simulink model "EMC_no_hand"  (R2015a)
settings: Solver=ode4  SolverMode=MultiTasking  StartTime=0.0  StopTime=inf  FixedStep=BKIN_STEP_TIME  RelTol=1e-3
StartFcn:
  |  warndlg('Dexterit-E models cannot run under simulation. Please compile your model and run it from within Dexterit-E.');set_param(bdroot,'SimulationCommand','stop')
model workspace (MAT data in the model file):
  BKIN_KINEMATIC_FRAME_SIZE = 400
  BKIN_STEP_TIME = 0.00025
  COLOR = 4
  COL_X = 1
  COL_Y = 2
  E_NO_EVENT = 0
  LOAD_X = 1
  LOAD_Y = 2
  MOVEMENT_DELAY = 3
  PATH_LENGTH = 1
  PATH_PERIOD = 2
  POST_TRIAL_DELAY = 4
  RADIUS = 3
  TRAJECTORY = 1
  TRAJECTORY_TYPE = 2
  TRIAL_END = 3
  TRIAL_MOVEMENT = 2
  TRIAL_RESET = 4
  TRIAL_START = 1
  X_POSITION = 1
  Y_POSITION = 2
  col_x = 1
  col_y = 2
  ANGULAR_THRESHOLD = 5
  GAZE_EXIT = 6
  START_REACHED = 7
  FIXATION_DURATION = 6
  TRACKING_TARGET_ROW = 7
  FEEDBACK_COLOR = 5
  CROSS_LOGICAL_RADIUS = 8
  DETECT_FIXATION = 8
  GAZE_IN_TARGET = 5
  START_STABILIZATION = 9
  HAND_IN_TARGET = 9
  BACKGROUND_LOAD = 10
  DIST_BETWEEN_TRAJ = 11
  STRAIGHT_PAUSE_TIME = 12
libraries: simulink x14, xpcrtudplib x12, xpcutilitieslib x10, xpcobsoletelib x8, slrtlib x2, ethercat x2, General x2, Video x2
(part 3 of 6)

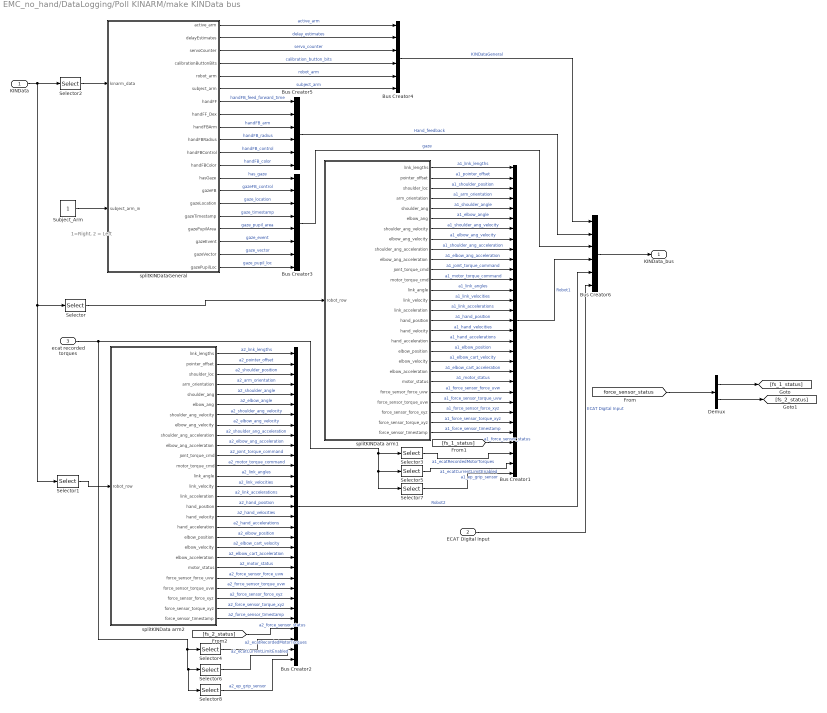
== system EMC_no_hand/DataLogging/Poll KINARM/make KINData bus ==
  note: 1=Right, 2 = Left
  KINData : Inport
  ECAT Digital Input : Inport  Port=2
  ecat recorded torques : Inport  Port=3
  Bus Creator1 : BusCreator  Inputs=31
  Bus Creator2 : BusCreator  Inputs=31
  Bus Creator3 : BusCreator  Inputs=8
  Bus Creator4 : BusCreator  Inputs=6
  Bus Creator5 : BusCreator  Inputs=6
  Bus Creator6 : BusCreator  Inputs=6
  Demux : Demux  Outputs=2
  Selector : Selector  NumberOfDimensions=2  InputPortWidth=3  IndexOptions=Index vector (dialog),Select all  Indices=[1],1  OutputSizes=1,1
  Selector1 : Selector  NumberOfDimensions=2  InputPortWidth=3  IndexOptions=Index vector (dialog),Select all  Indices=[2],1  OutputSizes=1,1
  Selector2 : Selector  NumberOfDimensions=2  InputPortWidth=3  IndexOptions=Index vector (dialog),Select all  Indices=[3],1  OutputSizes=1,1
  Selector3 : Selector  Indices=[1 2]
  Selector4 : Selector  Indices=[3, 4]
  Selector5 : Selector  Indices=[5 6]
  Selector6 : Selector  Indices=[7, 8]
  Selector7 : Selector  Indices=[9]
  Selector8 : Selector  Indices=[10]
  Subject_Arm : Constant
  splitKINData arm1 : MATLAB Function  TreatAsAtomicUnit=on
  splitKINData arm2 : MATLAB Function  TreatAsAtomicUnit=on
  splitKINDataGeneral : MATLAB Function  TreatAsAtomicUnit=on
  KINData_bus : Outport
  wires:
  splitKINDataGeneral/20(gazePupilLoc) -> Bus Creator3/8  "gaze_pupil_loc"
  splitKINDataGeneral/13(hasGaze) -> Bus Creator3/1  "has_gaze"
  splitKINDataGeneral/14(gazeFB) -> Bus Creator3/2  "gazeFB_control"
  splitKINDataGeneral/15(gazeLocation) -> Bus Creator3/3  "gaze_location"
  splitKINDataGeneral/16(gazeTimestamp) -> Bus Creator3/4  "gaze_timestamp"
  splitKINDataGeneral/17(gazePupilArea) -> Bus Creator3/5  "gaze_pupil_area"
  splitKINDataGeneral/18(gazeEvent) -> Bus Creator3/6  "gaze_event"
  splitKINData arm1/1(link_lengths) -> Bus Creator1/1  "a1_link_lengths"
  splitKINData arm1/2(pointer_offset) -> Bus Creator1/2  "a1_pointer_offset"
  splitKINData arm1/3(shoulder_loc) -> Bus Creator1/3  "a1_shoulder_position"
  splitKINData arm1/4(arm_orientation) -> Bus Creator1/4  "a1_arm_orientation"
  splitKINData arm1/5(shoulder_ang) -> Bus Creator1/5  "a1_shoulder_angle"
  splitKINData arm1/6(elbow_ang) -> Bus Creator1/6  "a1_elbow_angle"
  splitKINData arm1/7(shoulder_ang_velocity) -> Bus Creator1/7  "a1_shoulder_ang_velocity"
  splitKINData arm1/8(elbow_ang_velocity) -> Bus Creator1/8  "a1_elbow_ang_velocity"
  splitKINData arm1/11(joint_torque_cmd) -> Bus Creator1/11  "a1_joint_torque_command"
  splitKINData arm1/12(motor_torque_cmd) -> Bus Creator1/12  "a1_motor_torque_command"
  splitKINData arm1/13(link_angle) -> Bus Creator1/13  "a1_link_angles"
  splitKINData arm1/14(link_velocity) -> Bus Creator1/14  "a1_link_velocities"
  splitKINData arm1/15(link_acceleration) -> Bus Creator1/15  "a1_link_accelerations"
  splitKINData arm1/16(hand_position) -> Bus Creator1/16  "a1_hand_position"
  splitKINData arm1/17(hand_velocity) -> Bus Creator1/17  "a1_hand_velocities"
  splitKINData arm1/18(hand_acceleration) -> Bus Creator1/18  "a1_hand_accelerations"
  splitKINData arm1/22(motor_status) -> Bus Creator1/22  "a1_motor_status"
  splitKINData arm1/23(force_sensor_force_uvw) -> Bus Creator1/23  "a1_force_sensor_force_uvw"
  splitKINData arm1/24(force_sensor_torque_uvw) -> Bus Creator1/24  "a1_force_sensor_torque_uvw"
  splitKINData arm1/25(force_sensor_force_xyz) -> Bus Creator1/25  "a1_force_sensor_force_xyz"
  splitKINData arm1/26(force_sensor_torque_xyz) -> Bus Creator1/26  "a1_force_sensor_torque_xyz"
  splitKINData arm1/27(force_sensor_timestamp) -> Bus Creator1/27  "a1_force_sensor_timestamp"
  splitKINData arm2/1(link_lengths) -> Bus Creator2/1  "a2_link_lengths"
  splitKINData arm2/2(pointer_offset) -> Bus Creator2/2  "a2_pointer_offset"
  splitKINData arm2/3(shoulder_loc) -> Bus Creator2/3  "a2_shoulder_position"
  splitKINData arm2/4(arm_orientation) -> Bus Creator2/4  "a2_arm_orientation"
  splitKINData arm2/5(shoulder_ang) -> Bus Creator2/5  "a2_shoulder_angle"
  splitKINData arm2/6(elbow_ang) -> Bus Creator2/6  "a2_elbow_angle"
  splitKINData arm2/7(shoulder_ang_velocity) -> Bus Creator2/7  "a2_shoulder_ang_velocity"
  splitKINData arm2/11(joint_torque_cmd) -> Bus Creator2/11  "a2_joint_torque_command"
  splitKINData arm2/12(motor_torque_cmd) -> Bus Creator2/12  "a2_motor_torque_command"
  splitKINData arm2/13(link_angle) -> Bus Creator2/13  "a2_link_angles"
  splitKINData arm2/14(link_velocity) -> Bus Creator2/14  "a2_link_velocities"
  splitKINData arm2/15(link_acceleration) -> Bus Creator2/15  "a2_link_accelerations"
  splitKINData arm2/16(hand_position) -> Bus Creator2/16  "a2_hand_position"
  splitKINData arm2/17(hand_velocity) -> Bus Creator2/17  "a2_hand_velocities"
  splitKINData arm2/18(hand_acceleration) -> Bus Creator2/18  "a2_hand_accelerations"
  splitKINData arm2/22(motor_status) -> Bus Creator2/22  "a2_motor_status"
  splitKINData arm2/23(force_sensor_force_uvw) -> Bus Creator2/23  "a2_force_sensor_force_uvw"
  splitKINData arm2/24(force_sensor_torque_uvw) -> Bus Creator2/24  "a2_force_sensor_torque_uvw"
  splitKINData arm2/25(force_sensor_force_xyz) -> Bus Creator2/25  "a2_force_sensor_force_xyz"
  splitKINData arm2/26(force_sensor_torque_xyz) -> Bus Creator2/26  "a2_force_sensor_torque_xyz"
  splitKINData arm2/27(force_sensor_timestamp) -> Bus Creator2/27  "a2_force_sensor_timestamp"
  Selector/1 -> splitKINData arm1/1(robot_row)
  Selector1/1 -> splitKINData arm2/1(robot_row)
  splitKINDataGeneral/1(active_arm) -> Bus Creator4/1  "active_arm"
  splitKINDataGeneral/2(delayEstimates) -> Bus Creator4/2  "delay_estimates"
  splitKINDataGeneral/3(servoCounter) -> Bus Creator4/3  "servo_counter"
  splitKINDataGeneral/4(calibrationButtonBits) -> Bus Creator4/4  "calibration_button_bits"
  splitKINDataGeneral/7(handFF) -> Bus Creator5/1  "handFB_feed_forward_time"
  splitKINDataGeneral/9(handFBArm) -> Bus Creator5/3  "handFB_arm"
  splitKINDataGeneral/10(handFBRadius) -> Bus Creator5/4  "handFB_radius"
  splitKINDataGeneral/11(handFBControl) -> Bus Creator5/5  "handFB_control"
  splitKINDataGeneral/12(handFBColor) -> Bus Creator5/6  "handFB_color"
  Bus Creator4/1 -> Bus Creator6/1  "KINDataGeneral"
  Bus Creator5/1 -> Bus Creator6/2  "Hand_feedback"
  Bus Creator3/1 -> Bus Creator6/3  "gaze"
  Bus Creator1/1 -> Bus Creator6/4  "Robot1"
  Bus Creator2/1 -> Bus Creator6/5  "Robot2"
  KINData/1 -> Selector1/1, Selector/1, Selector2/1
  Bus Creator6/1 -> KINData_bus/1
  Selector2/1 -> splitKINDataGeneral/1(kinarm_data)
  ECAT Digital Input/1 -> Bus Creator6/6  "ECAT Digital Input"
  ecat recorded torques/1 -> Selector7/1, Selector5/1, Selector3/1, Selector4/1, Selector8/1, Selector6/1
  Selector3/1 -> Bus Creator1/29  "a1_ecatRecordedMotorTorques"
  Selector4/1 -> Bus Creator2/29  "a2_ecatRecordedMotorTorques"
  Selector5/1 -> Bus Creator1/30  "a1_ecatCurrentLimitEnabled"
  Selector6/1 -> Bus Creator2/30  "a2_ecatCurrentLimitEnabled"
  splitKINDataGeneral/8(handFF_Dex) -> Bus Creator5/2
  splitKINDataGeneral/19(gazeVector) -> Bus Creator3/7  "gaze_vector"
  [force_sensor_status] -> Demux/1
  Demux/1 -> [fs_1_status]
  Demux/2 -> [fs_2_status]
  [fs_1_status] -> Bus Creator1/28  "a1_force_sensor_status"
  [fs_2_status] -> Bus Creator2/28  "a2_force_sensor_status"
  splitKINData arm1/9(shoulder_ang_acceleration) -> Bus Creator1/9  "a1_shoulder_ang_acceleration"
  splitKINData arm1/10(elbow_ang_acceleration) -> Bus Creator1/10  "a1_elbow_ang_acceleration"
  splitKINData arm1/19(elbow_position) -> Bus Creator1/19  "a1_elbow_position"
  splitKINData arm1/20(elbow_velocity) -> Bus Creator1/20  "a1_elbow_cart_velocity"
  splitKINData arm1/21(elbow_acceleration) -> Bus Creator1/21  "a1_elbow_cart_acceleration"
  splitKINData arm2/10(elbow_ang_acceleration) -> Bus Creator2/10  "a2_elbow_ang_acceleration"
  splitKINData arm2/21(elbow_acceleration) -> Bus Creator2/21  "a2_elbow_cart_acceleration"
  splitKINData arm2/20(elbow_velocity) -> Bus Creator2/20  "a2_elbow_cart_velocity"
  splitKINData arm2/19(elbow_position) -> Bus Creator2/19  "a2_elbow_position"
  splitKINData arm2/8(elbow_ang_velocity) -> Bus Creator2/8  "a2_elbow_ang_velocity"
  splitKINData arm2/9(shoulder_ang_acceleration) -> Bus Creator2/9  "a2_shoulder_ang_acceleration"
  Selector7/1 -> Bus Creator1/31  "a1_ep_grip_sensor"
  Selector8/1 -> Bus Creator2/31  "a2_ep_grip_sensor"
  splitKINDataGeneral/6(subject_arm) -> Bus Creator4/6  "subject_arm"
  splitKINDataGeneral/5(robot_arm) -> Bus Creator4/5  "robot_arm"
  Subject_Arm/1 -> splitKINDataGeneral/2(subject_arm_in)

== system EMC_no_hand/DataLogging/Poll KINARM/split_primary ==
  primary data : Inport
  Bus Creator1 : BusCreator  Inputs=3
  Bus Creator2 : BusCreator  Inputs=2
  Bus Creator4 : BusCreator  Inputs=3
  Selector1 : Selector  NumberOfDimensions=2  InputPortWidth=3  IndexOptions=Index vector (dialog),Select all  Indices=[2],1  OutputSizes=1,1
  Selector2 : Selector  NumberOfDimensions=2  InputPortWidth=3  IndexOptions=Index vector (dialog),Select all  Indices=[1],1  OutputSizes=1,1
  split_primary : MATLAB Function  TreatAsAtomicUnit=on
  split_primary1 : MATLAB Function  TreatAsAtomicUnit=on
  primary_data_bus : Outport
  wires:
  split_primary/1(link_angles) -> Bus Creator4/1  "a1_link_angles"
  split_primary/2(link_velocities) -> Bus Creator4/2  "a1_link_velocities"
  split_primary/3(link_acceleration) -> Bus Creator4/3  "a1_link_accelerations"
  primary data/1 -> Selector2/1, Selector1/1
  Selector2/1 -> split_primary/1(primary_data)
  split_primary1/1(link_angles) -> Bus Creator1/1  "a2_link_angles"
  split_primary1/2(link_velocities) -> Bus Creator1/2  "a2_link_velocities"
  split_primary1/3(link_acceleration) -> Bus Creator1/3  "a2_link_accelerations"
  Selector1/1 -> split_primary1/1(primary_data)
  Bus Creator4/1 -> Bus Creator2/1  "robot1"
  Bus Creator1/1 -> Bus Creator2/2  "robot2"
  Bus Creator2/1 -> primary_data_bus/1

== system EMC_no_hand/DataLogging/apply loads/apply pmac loads ==
  Force scale : Inport
  Torques : Inport  Port=2
  Robot 1 motor parms : Inport  Port=3
  Robot 2 motor parms : Inport  Port=4
  Enable : EnablePort
  Bus Selector : BusSelector  OutputSignals=R1.Arm Orientation,R1.M1 orientation,R1.M2 Orientation,R1.M1 Gear Ratio,R1.M2 Gear Ratio,torque constant  OutputAsBus=on
  Bus Selector1 : BusSelector  OutputSignals=R2.Arm Orientation,R2.M1 orientation,R2.M2 Orientation,R2.M1 Gear Ratio,R2.M2 Gear Ratio,torque constant  OutputAsBus=on
  Bus to Vector : BusToVector
  Bus to Vector1 : BusToVector
  Data Type Conversion : DataTypeConversion
  Data Type Conversion1 : DataTypeConversion
  Data Type Conversion6 : DataTypeConversion  OutDataTypeStr=single
  Product : Product  RndMeth=Zero
  S-Function1 : S-Function  FunctionName=mcc_apply_loads
  wires:
  Torques/1 -> Product/1
  Data Type Conversion6/1 -> S-Function1/1
  Product/1 -> Data Type Conversion6/1
  Bus to Vector1/1 -> Data Type Conversion1/1
  Bus to Vector/1 -> Data Type Conversion/1
  Force scale/1 -> Product/2
  Robot 2 motor parms/1 -> Bus Selector1/1
  Data Type Conversion/1 -> S-Function1/2
  Data Type Conversion1/1 -> S-Function1/3
  Robot 1 motor parms/1 -> Bus Selector/1
  Bus Selector/1 -> Bus to Vector/1
  Bus Selector1/1 -> Bus to Vector1/1

== system EMC_no_hand/DataLogging/create_lab_info/Subsystem ==
  Bus Creator : BusCreator  Inputs=5
  Bus Creator1 : BusCreator  Inputs=5
  Bus Selector : BusSelector  OutputSignals=R1.Arm Orientation,R1.Has Secondary Enc,R1Info.isEP
  Bus Selector1 : BusSelector  OutputSignals=R2.Arm Orientation,R2.Has Secondary Enc,R2Info.isEP
  Demux : Demux  Outputs=2
  MATLAB Function : MATLAB Function  TreatAsAtomicUnit=on
  MATLAB Function1 : MATLAB Function  TreatAsAtomicUnit=on
  robot_1_info : Outport
  robot_2_info : Outport  Port=2
  wires:
  Bus Selector/1 -> MATLAB Function/1(orientation)  "<Arm Orientation>"
  [robot1_motor_parameters] -> Bus Selector/1
  Bus Selector/3 -> Bus Creator/3, MATLAB Function/3(isEP)  "<isEP>"
  Bus Selector/2 -> MATLAB Function/2(has_secondary)  "<Has Secondary Enc>"
  MATLAB Function/1(is_right_arm) -> Bus Creator/1
  MATLAB Function/2(isExo) -> Bus Creator/2
  MATLAB Function/3(has_high_res_encoders) -> Bus Creator/4
  Bus Creator/1 -> robot_1_info/1
  Bus Selector1/1 -> MATLAB Function1/1(orientation)  "<Arm Orientation>"
  [robot2_motor_parameters] -> Bus Selector1/1
  Bus Selector1/3 -> Bus Creator1/3, MATLAB Function1/3(isEP)  "<isEP>"
  Bus Selector1/2 -> MATLAB Function1/2(has_secondary)  "<Has Secondary Enc>"
  MATLAB Function1/1(is_right_arm) -> Bus Creator1/1
  MATLAB Function1/2(isExo) -> Bus Creator1/2
  MATLAB Function1/3(has_high_res_encoders) -> Bus Creator1/4
  Bus Creator1/1 -> robot_2_info/1
  [has_force_sensor] -> Demux/1
  Demux/1 -> Bus Creator/5  "has_force_torque_sensor"
  Demux/2 -> Bus Creator1/5  "has_force_torque_sensor"

== system EMC_no_hand/DataLogging/monitor torques/delay ==
  command : Inport
  Delay : Delay  DelayLength=6
  butterworth_2nd_order_250hz : Constant  Value=[3.338387406e+01 -0.5740619151 1.4542435863]
  filter : MATLAB Function  TreatAsAtomicUnit=on  SystemSampleTime=BKIN_STEP_TIME
  command_delayed : Outport
  wires:
  filter/1(filteredVals) -> Delay/1
  butterworth_2nd_order_250hz/1 -> filter/2(filterConsts)
  Delay/1 -> command_delayed/1
  command/1 -> filter/1(data)

== system EMC_no_hand/DataLogging/Network Transfer Subsystem/Data Packing Subsystem/Counter ==
  Constant : Constant
  Sum : Sum  Inputs=|++  SaturateOnIntegerOverflow=on
  Unit Delay : UnitDelay  SampleTime=-1
  count : Outport
  wires:
  Constant/1 -> Sum/2
  Sum/1 -> Unit Delay/1, count/1
  Unit Delay/1 -> Sum/1

== system EMC_no_hand/DataLogging/Poll KINARM/Force Sensor Control/Force Sensor 1 Subsystem ==
  Force Sensor 1 Present : Inport
  Byte Reversal : xpcutilitieslib/Byte Reversal   numInp=1
  Byte Reversal1 : xpcutilitieslib/Byte Reversal   numInp=1
  Constant : Constant  Value=zeros(1, 7);  OutDataTypeStr=double
  Create timestamp : MATLAB Function  TreatAsAtomicUnit=on
  Data Type Conversion : DataTypeConversion
  Detect Change : simulink/Logic and Bit Operations/Detect Change  vinit=-1  InputProcessing=Inherited  OutDataTypeStr=uint8
  If Action Subsystem : Subsystem  TreatAsAtomicUnit=on
  Mux : Mux  Inputs=2
  Receive from Robot 1 Force Sensor : xpcrtudplib/Legacy UDP/Receive   ipAddress=192.168.0.10  ipPort=51000  width=36  vblLen=off  sampletime=BKIN_STEP_TIME
  Selector : Selector  InputPortWidth=3  Indices=3
  Switch : Switch  Criteria=u2 > Threshold
  Terminator : Terminator
  Unpack : xpcobsoletelib/Utilities/Unpack   dimensions={3, 6}  datatypes={'uint32', 'int32'}  byteAlign=1
  Out1 : Outport
  status : Outport  Port=2
  wires:
  Receive from Robot 1 Force Sensor/1 -> Unpack/1
  Receive from Robot 1 Force Sensor/2 -> Terminator/1
  Force Sensor 1 Present/1 -> Switch/2, If Action Subsystem/1(In1), Detect Change/1
  Constant/1 -> Switch/3
  Switch/1 -> Out1/1
  Unpack/2 -> Byte Reversal/1
  Unpack/1 -> Byte Reversal1/1
  Byte Reversal/1 -> Data Type Conversion/1
  Detect Change/1 -> If Action Subsystem/Enable
  Create timestamp/1(timestamp_out) -> Mux/2
  Data Type Conversion/1 -> Mux/1
  Mux/1 -> Switch/1
  Byte Reversal1/1 -> Selector/1, Create timestamp/1(times_in)
  Selector/1 -> status/1

== system EMC_no_hand/DataLogging/Poll KINARM/Force Sensor Control/Force Sensor 2 Subsystem ==
  Force Sensor 2 Present : Inport
  Byte Reversal : xpcutilitieslib/Byte Reversal   numInp=1
  Byte Reversal1 : xpcutilitieslib/Byte Reversal   numInp=1
  Constant1 : Constant  Value=zeros(1, 7);  OutDataTypeStr=double
  Create timestamp : MATLAB Function  TreatAsAtomicUnit=on
  Data Transfer Start Subsystem : Subsystem  TreatAsAtomicUnit=on
  Data Type Conversion1 : DataTypeConversion
  Detect Change : simulink/Logic and Bit Operations/Detect Change  vinit=-1  InputProcessing=Inherited  OutDataTypeStr=uint8
  Mux : Mux  Inputs=2
  Receive from Robot 2 Force Sensor : xpcrtudplib/Legacy UDP/Receive   ipAddress=192.168.0.11  ipPort=51001  width=36  vblLen=off  sampletime=BKIN_STEP_TIME
  Selector : Selector  InputPortWidth=3  Indices=3
  Switch1 : Switch  Criteria=u2 > Threshold
  Terminator1 : Terminator
  Unpack1 : xpcobsoletelib/Utilities/Unpack   dimensions={3, 6}  datatypes={'uint32', 'int32'}  byteAlign=1
  Out1 : Outport
  status : Outport  Port=2
  wires:
  Receive from Robot 2 Force Sensor/1 -> Unpack1/1
  Receive from Robot 2 Force Sensor/2 -> Terminator1/1
  Force Sensor 2 Present/1 -> Data Transfer Start Subsystem/1(In2), Detect Change/1, Switch1/2
  Constant1/1 -> Switch1/3
  Switch1/1 -> Out1/1
  Unpack1/2 -> Byte Reversal/1
  Byte Reversal/1 -> Data Type Conversion1/1
  Detect Change/1 -> Data Transfer Start Subsystem/Enable
  Unpack1/1 -> Byte Reversal1/1
  Data Type Conversion1/1 -> Mux/1
  Create timestamp/1(timestamp_out) -> Mux/2
  Mux/1 -> Switch1/1
  Byte Reversal1/1 -> Selector/1, Create timestamp/1(times_in)
  Selector/1 -> status/1

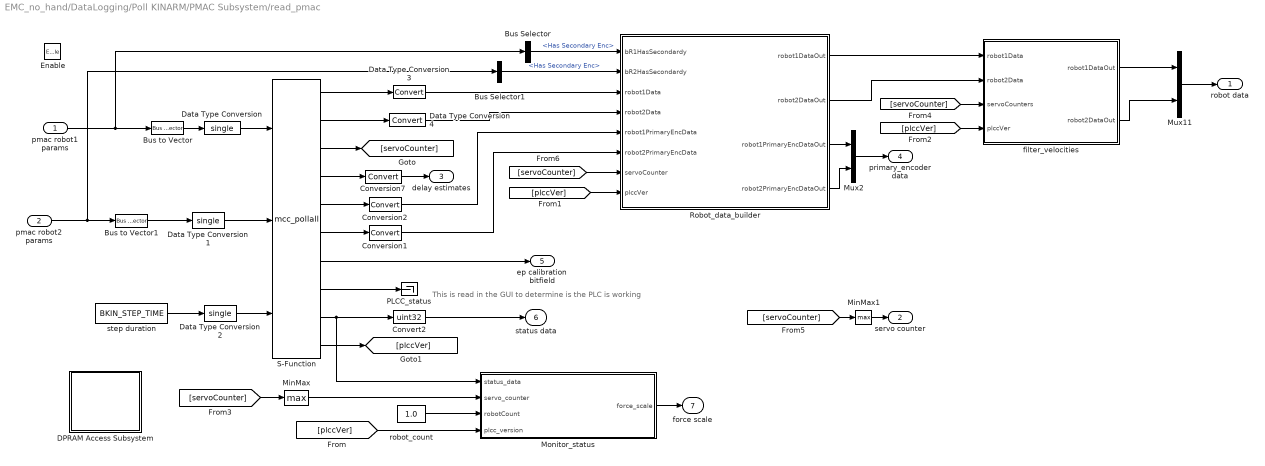
== system EMC_no_hand/DataLogging/Poll KINARM/PMAC Subsystem/read_pmac ==
  note: This is read in the GUI to determine is the PLC is working
  pmac robot1 params : Inport
  pmac robot2 params : Inport  Port=2
  Enable : EnablePort
  Bus Selector : BusSelector  OutputSignals=R1.Has Secondary Enc
  Bus Selector1 : BusSelector  OutputSignals=R2.Has Secondary Enc
  Bus to Vector : BusToVector
  Bus to Vector1 : BusToVector
  Conversion1 : DataTypeConversion
  Conversion2 : DataTypeConversion
  Conversion7 : DataTypeConversion
  Convert2 : DataTypeConversion  OutDataTypeStr=uint32
  DPRAM Access Subsystem : Subsystem
  Data Type Conversion : DataTypeConversion  OutDataTypeStr=single
  Data Type Conversion1 : DataTypeConversion  OutDataTypeStr=single
  Data Type Conversion2 : DataTypeConversion  OutDataTypeStr=single
  Data Type Conversion3 : DataTypeConversion
  Data Type Conversion4 : DataTypeConversion
  MinMax : MinMax  Function=max
  MinMax1 : MinMax  Function=max
  Monitor_status : MATLAB Function  TreatAsAtomicUnit=on  SystemSampleTime=BKIN_STEP_TIME
  Mux11 : Mux  Inputs=2
  Mux2 : Mux  Inputs=2
  PLCC_status : Terminator
  Robot_data_builder : MATLAB Function  TreatAsAtomicUnit=on
  S-Function : S-Function  FunctionName=mcc_pollall
  filter_velocities : MATLAB Function  TreatAsAtomicUnit=on
  robot_count : Constant  Value=1.0
  step duration : Constant  Value=BKIN_STEP_TIME  OutDataTypeStr=double
  robot data : Outport
  servo counter : Outport  Port=2
  delay estimates : Outport  Port=3
  primary_encoder data : Outport  Port=4
  ep calibration bitfield : Outport  Port=5
  status data : Outport  Port=6
  force scale : Outport  Port=7
  wires:
  MinMax/1 -> Monitor_status/2(servo_counter)
  pmac robot1 params/1 -> Bus to Vector/1, Bus Selector/1
  pmac robot2 params/1 -> Bus to Vector1/1, Bus Selector1/1
  Mux11/1 -> robot data/1
  Conversion7/1 -> delay estimates/1
  robot_count/1 -> Monitor_status/3(robotCount)
  Data Type Conversion4/1 -> Robot_data_builder/4(robot2Data)
  Data Type Conversion3/1 -> Robot_data_builder/3(robot1Data)
  Robot_data_builder/3(robot1PrimaryEncDataOut) -> Mux2/1
  Robot_data_builder/4(robot2PrimaryEncDataOut) -> Mux2/2
  Mux2/1 -> primary_encoder data/1
  Conversion2/1 -> Robot_data_builder/5(robot1PrimaryEncData)
  Conversion1/1 -> Robot_data_builder/6(robot2PrimaryEncData)
  S-Function/4 -> Conversion7/1
  S-Function/5 -> Conversion2/1
  step duration/1 -> Data Type Conversion2/1
  Data Type Conversion/1 -> S-Function/1
  S-Function/9 -> Monitor_status/1(status_data), Convert2/1
  S-Function/1 -> Data Type Conversion3/1
  Data Type Conversion1/1 -> S-Function/2
  Convert2/1 -> status data/1
  S-Function/8 -> PLCC_status/1
  S-Function/6 -> Conversion1/1
  S-Function/7 -> ep calibration bitfield/1
  S-Function/2 -> Data Type Conversion4/1
  Monitor_status/1(force_scale) -> force scale/1
  Bus to Vector/1 -> Data Type Conversion/1
  Bus to Vector1/1 -> Data Type Conversion1/1
  Bus Selector/1 -> Robot_data_builder/1(bR1HasSecondardy)  "<Has Secondary Enc>"
  Bus Selector1/1 -> Robot_data_builder/2(bR2HasSecondardy)  "<Has Secondary Enc>"
  Data Type Conversion2/1 -> S-Function/3
  Robot_data_builder/1(robot1DataOut) -> filter_velocities/1(robot1Data)
  Robot_data_builder/2(robot2DataOut) -> filter_velocities/2(robot2Data)
  S-Function/3 -> [servoCounter]
  S-Function/10 -> [plccVer]
  [plccVer] -> Monitor_status/4(plcc_version)
  [plccVer] -> Robot_data_builder/8(plccVer)
  [plccVer] -> filter_velocities/4(plccVer)
  [servoCounter] -> MinMax/1
  [servoCounter] -> filter_velocities/3(servoCounters)
  filter_velocities/1(robot1DataOut) -> Mux11/1
  filter_velocities/2(robot2DataOut) -> Mux11/2
  [servoCounter] -> MinMax1/1
  [servoCounter] -> Robot_data_builder/7(servoCounter)
  MinMax1/1 -> servo counter/1

== system EMC_no_hand/DataLogging/Poll KINARM/PMAC Subsystem/update settings ==
  Kinematics : Inport
  Servo counter : Inport  Port=2
  delay estimates : Inport  Port=3
  primry enc data : Inport  Port=4
  EP Calibration Button : Inport  Port=5
  Robot status : Inport  Port=6
  function : TriggerPort  TriggerType=function-call
  Data Store Write1 : DataStoreWrite  DataStoreName=Kinematics
  Data Store Write2 : DataStoreWrite  DataStoreName=ServoUpdate
  Data Store Write3 : DataStoreWrite  DataStoreName=DelayEstimates
  Data Store Write4 : DataStoreWrite  DataStoreName=PrimaryEncoderData
  Data Store Write5 : DataStoreWrite  DataStoreName=CalibrationButton
  Data Store Write7 : DataStoreWrite  DataStoreName=SystemStatus
  update status format : MATLAB Function  TreatAsAtomicUnit=on
  wires:
  Kinematics/1 -> Data Store Write1/1
  Servo counter/1 -> Data Store Write2/1
  delay estimates/1 -> Data Store Write3/1
  primry enc data/1 -> Data Store Write4/1
  EP Calibration Button/1 -> Data Store Write5/1
  update status format/1(outStatus) -> Data Store Write7/1
  Robot status/1 -> update status format/1(pmacStatus)

== system EMC_no_hand/DataLogging/Poll KINARM/bkin_internal_testing/Data receive ==
  Enable : EnablePort
  Constant : Constant  Value=0  OutDataTypeStr=uint32
  Constant1 : Constant  Value=zeros(7, 1)  OutDataTypeStr=uint32
  Counter Free-Running : simulink/Sources/Counter Free-Running  NumBits=32  tsamp=BKIN_STEP_TIME
  Data Type Conversion : DataTypeConversion
  Data Type Conversion1 : DataTypeConversion
  Data Type Conversion2 : DataTypeConversion
  MATLAB Function : MATLAB Function  TreatAsAtomicUnit=on
  Receive : xpcrtudplib/Legacy UDP/Receive   ipAddress=192.168.0.1  ipPort=50050  width=16  vblLen=on  sampletime=BKIN_STEP_TIME
  Unpack : xpcobsoletelib/Utilities/Unpack   dimensions={2, 2}  datatypes={'single', 'single'}  byteAlign=1
  Kinematics : Outport
  primary enc : Outport  Port=2
  servo counter : Outport  Port=3  InitialOutput=0
  EP calibration btn : Outport  Port=4  InitialOutput=uint32(0)
  Status bits : Outport  Port=5  InitialOutput=zeros(7,1, 'uint32')
  wires:
  Receive/1 -> Unpack/1
  Counter Free-Running/1 -> Data Type Conversion2/1, servo counter/1
  Constant/1 -> EP calibration btn/1
  Constant1/1 -> Status bits/1
  MATLAB Function/1(kinematics) -> Kinematics/1
  MATLAB Function/2(primary) -> primary enc/1
  Receive/2 -> MATLAB Function/3(is_new_data)
  Unpack/1 -> Data Type Conversion/1
  Unpack/2 -> Data Type Conversion1/1
  Data Type Conversion/1 -> MATLAB Function/1(r1ShoElb)
  Data Type Conversion1/1 -> MATLAB Function/2(r2ShoElb)
  Data Type Conversion2/1 -> MATLAB Function/4(clock_tick)

== system EMC_no_hand/DataLogging/Poll KINARM/bkin_internal_testing/Data write ==
  Kinematics : Inport
  primry enc data : Inport  Port=2
  Servo counter : Inport  Port=3
  EP Calibration Button : Inport  Port=4
  Robot status : Inport  Port=5
  function : TriggerPort  TriggerType=function-call
  Constant : Constant  Value=zeros(4, 1)
  Data Store Write1 : DataStoreWrite  DataStoreName=Kinematics
  Data Store Write2 : DataStoreWrite  DataStoreName=ServoUpdate
  Data Store Write3 : DataStoreWrite  DataStoreName=DelayEstimates
  Data Store Write4 : DataStoreWrite  DataStoreName=PrimaryEncoderData
  Data Store Write5 : DataStoreWrite  DataStoreName=CalibrationButton
  Data Store Write7 : DataStoreWrite  DataStoreName=SystemStatus
  wires:
  Kinematics/1 -> Data Store Write1/1
  Servo counter/1 -> Data Store Write2/1
  Constant/1 -> Data Store Write3/1
  primry enc data/1 -> Data Store Write4/1
  EP Calibration Button/1 -> Data Store Write5/1
  Robot status/1 -> Data Store Write7/1

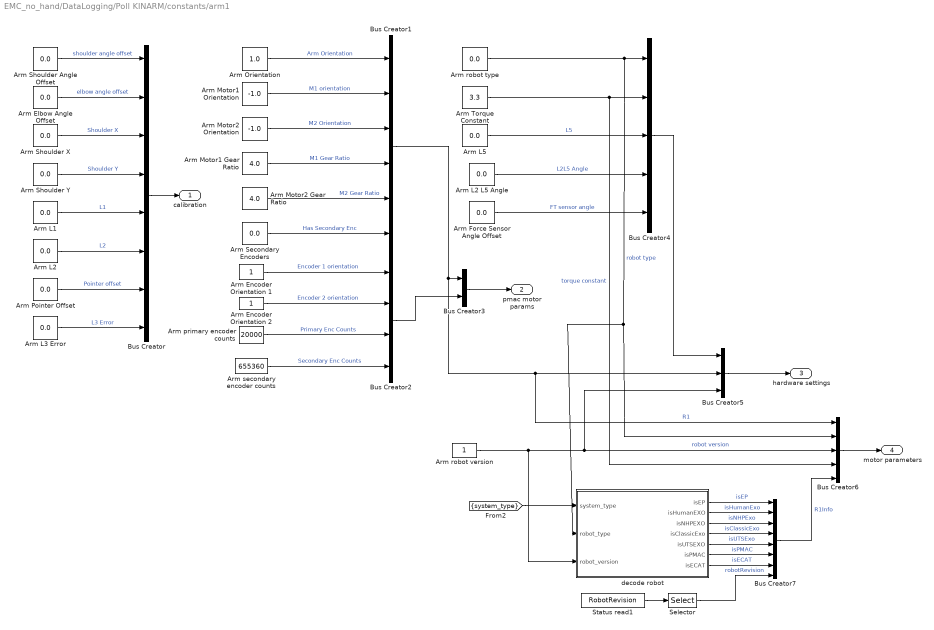
== system EMC_no_hand/DataLogging/Poll KINARM/constants/arm1 ==
  Arm Elbow Angle Offset : Constant  Value=0.0  SampleTime=BKIN_STEP_TIME
  Arm Encoder Orientation 1 : Constant
  Arm Encoder Orientation 2 : Constant
  Arm Force Sensor Angle Offset : Constant  Value=0.0
  Arm L1 : Constant  Value=0.0  SampleTime=BKIN_STEP_TIME
  Arm L2 : Constant  Value=0.0  SampleTime=BKIN_STEP_TIME
  Arm L2 L5 Angle : Constant  Value=0.0
  Arm L3 Error : Constant  Value=0.0  SampleTime=BKIN_STEP_TIME
  Arm L5 : Constant  Value=0.0
  Arm Motor1 Gear Ratio : Constant  Value=4.0
  Arm Motor1 Orientation : Constant  Value=-1.0
  Arm Motor2 Gear Ratio : Constant  Value=4.0
  Arm Motor2 Orientation : Constant  Value=-1.0
  Arm Orientation : Constant  Value=1.0
  Arm Pointer Offset : Constant  Value=0.0  SampleTime=BKIN_STEP_TIME
  Arm Secondary Encoders : Constant  Value=0.0
  Arm Shoulder Angle Offset : Constant  Value=0.0  SampleTime=BKIN_STEP_TIME
  Arm Shoulder X : Constant  Value=0.0  SampleTime=BKIN_STEP_TIME
  Arm Shoulder Y : Constant  Value=0.0  SampleTime=BKIN_STEP_TIME
  Arm Torque Constant : Constant  Value=3.3
  Arm primary encoder counts : Constant  Value=20000
  Arm robot type : Constant  Value=0.0
  Arm robot version : Constant
  Arm secondary encoder counts : Constant  Value=655360
  Bus Creator : BusCreator  Inputs=8
  Bus Creator1 : BusCreator  Inputs=6
  Bus Creator2 : BusCreator
  Bus Creator3 : BusCreator  Inputs=2
  Bus Creator4 : BusCreator  Inputs=5
  Bus Creator5 : BusCreator  Inputs=3
  Bus Creator6 : BusCreator  Inputs=5
  Bus Creator7 : BusCreator  Inputs=8
  Selector : Selector  Indices=[1]
  Status read1 : DataStoreRead  DataStoreName=RobotRevision  SampleTime=BKIN_STEP_TIME
  decode robot : MATLAB Function  TreatAsAtomicUnit=on
  calibration : Outport
  pmac motor params : Outport  Port=2
  hardware settings : Outport  Port=3
  motor parameters : Outport  Port=4
  wires:
  Arm secondary encoder counts/1 -> Bus Creator2/4  "Secondary Enc Counts"
  Arm primary encoder counts/1 -> Bus Creator2/3  "Primary Enc Counts"
  Arm Orientation/1 -> Bus Creator1/1  "Arm Orientation"
  Arm Motor1 Orientation/1 -> Bus Creator1/2  "M1 orientation"
  Arm Motor2 Orientation/1 -> Bus Creator1/3  "M2 Orientation"
  Arm Motor1 Gear Ratio/1 -> Bus Creator1/4  "M1 Gear Ratio"
  Arm Motor2 Gear Ratio/1 -> Bus Creator1/5  "M2 Gear Ratio"
  Arm Secondary Encoders/1 -> Bus Creator1/6  "Has Secondary Enc"
  Arm robot type/1 -> Bus Creator4/1, Bus Creator6/2, decode robot/2(robot_type)  "robot type"
  Arm Torque Constant/1 -> Bus Creator4/2, Bus Creator6/4  "torque constant"
  Arm L5/1 -> Bus Creator4/3  "L5"
  Arm L2 L5 Angle/1 -> Bus Creator4/4  "L2L5 Angle"
  Bus Creator4/1 -> Bus Creator5/1
  Arm Force Sensor Angle Offset/1 -> Bus Creator4/5  "FT sensor angle"
  Arm Encoder Orientation 1/1 -> Bus Creator2/1  "Encoder 1 orientation"
  Arm Encoder Orientation 2/1 -> Bus Creator2/2  "Encoder 2 orientation"
  Bus Creator2/1 -> Bus Creator3/2
  Bus Creator3/1 -> pmac motor params/1
  Bus Creator5/1 -> hardware settings/1
  Bus Creator6/1 -> motor parameters/1
  Arm Shoulder Angle Offset/1 -> Bus Creator/1  "shoulder angle offset"
  Arm Elbow Angle Offset/1 -> Bus Creator/2  "elbow angle offset"
  Arm Shoulder X/1 -> Bus Creator/3  "Shoulder X"
  Arm Shoulder Y/1 -> Bus Creator/4  "Shoulder Y"
  Arm L1/1 -> Bus Creator/5  "L1"
  Arm L2/1 -> Bus Creator/6  "L2"
  Arm Pointer Offset/1 -> Bus Creator/7  "Pointer offset"
  Arm L3 Error/1 -> Bus Creator/8  "L3 Error"
  Bus Creator/1 -> calibration/1
  Bus Creator1/1 -> Bus Creator6/1, Bus Creator5/2, Bus Creator3/1  "R1"
  Arm robot version/1 -> Bus Creator6/3, Bus Creator5/3, decode robot/3(robot_version)  "robot version"
  [system_type] -> decode robot/1(system_type)
  decode robot/1(isEP) -> Bus Creator7/1  "isEP"
  decode robot/2(isHumanEXO) -> Bus Creator7/2  "isHumanExo"
  decode robot/3(isNHPEXO) -> Bus Creator7/3  "isNHPExo"
  decode robot/4(isClassicExo) -> Bus Creator7/4  "isClassicExo"
  decode robot/5(isUTSEXO) -> Bus Creator7/5  "isUTSExo"
  decode robot/6(isPMAC) -> Bus Creator7/6  "isPMAC"
  decode robot/7(isECAT) -> Bus Creator7/7  "isECAT"
  Bus Creator7/1 -> Bus Creator6/5  "R1Info"
  Status read1/1 -> Selector/1
  Selector/1 -> Bus Creator7/8  "robotRevision"

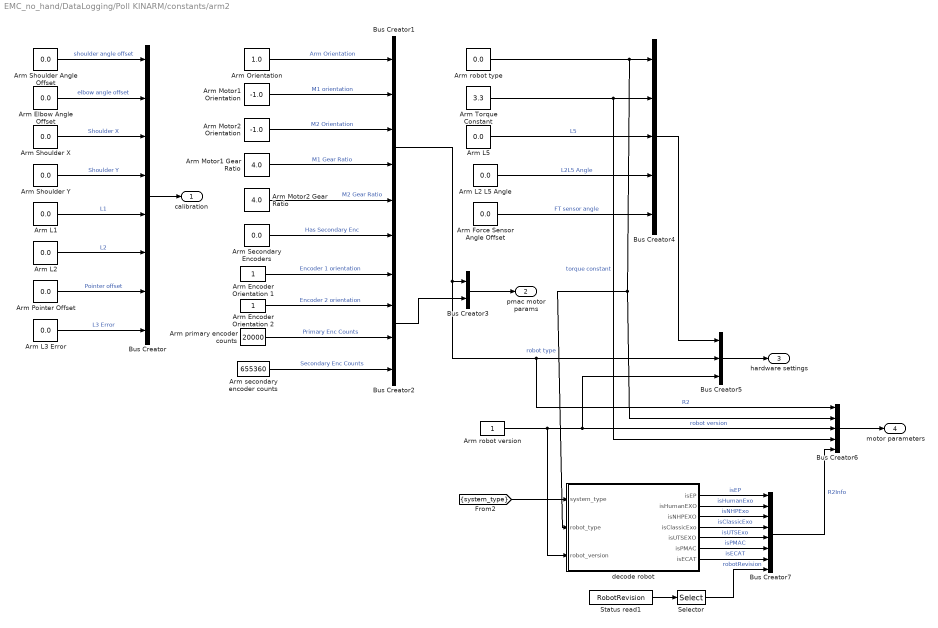
== system EMC_no_hand/DataLogging/Poll KINARM/constants/arm2 ==
  Arm Elbow Angle Offset : Constant  Value=0.0
  Arm Encoder Orientation 1 : Constant
  Arm Encoder Orientation 2 : Constant
  Arm Force Sensor Angle Offset : Constant  Value=0.0
  Arm L1 : Constant  Value=0.0
  Arm L2 : Constant  Value=0.0
  Arm L2 L5 Angle : Constant  Value=0.0
  Arm L3 Error : Constant  Value=0.0
  Arm L5 : Constant  Value=0.0
  Arm Motor1 Gear Ratio : Constant  Value=4.0
  Arm Motor1 Orientation : Constant  Value=-1.0
  Arm Motor2 Gear Ratio : Constant  Value=4.0
  Arm Motor2 Orientation : Constant  Value=-1.0
  Arm Orientation : Constant  Value=1.0
  Arm Pointer Offset : Constant  Value=0.0
  Arm Secondary Encoders : Constant  Value=0.0
  Arm Shoulder Angle Offset : Constant  Value=0.0
  Arm Shoulder X : Constant  Value=0.0
  Arm Shoulder Y : Constant  Value=0.0
  Arm Torque Constant : Constant  Value=3.3
  Arm primary encoder counts : Constant  Value=20000
  Arm robot type : Constant  Value=0.0
  Arm robot version : Constant
  Arm secondary encoder counts : Constant  Value=655360
  Bus Creator : BusCreator  Inputs=8
  Bus Creator1 : BusCreator  Inputs=6
  Bus Creator2 : BusCreator
  Bus Creator3 : BusCreator  Inputs=2
  Bus Creator4 : BusCreator  Inputs=5
  Bus Creator5 : BusCreator  Inputs=3
  Bus Creator6 : BusCreator  Inputs=5
  Bus Creator7 : BusCreator  Inputs=8
  Selector : Selector  Indices=[2]
  Status read1 : DataStoreRead  DataStoreName=RobotRevision  SampleTime=BKIN_STEP_TIME
  decode robot : MATLAB Function  TreatAsAtomicUnit=on
  calibration : Outport
  pmac motor params : Outport  Port=2
  hardware settings : Outport  Port=3
  motor parameters : Outport  Port=4
  wires:
  Arm secondary encoder counts/1 -> Bus Creator2/4  "Secondary Enc Counts"
  Arm primary encoder counts/1 -> Bus Creator2/3  "Primary Enc Counts"
  Arm Orientation/1 -> Bus Creator1/1  "Arm Orientation"
  Arm Motor1 Orientation/1 -> Bus Creator1/2  "M1 orientation"
  Arm Motor2 Orientation/1 -> Bus Creator1/3  "M2 Orientation"
  Arm Motor1 Gear Ratio/1 -> Bus Creator1/4  "M1 Gear Ratio"
  Arm Motor2 Gear Ratio/1 -> Bus Creator1/5  "M2 Gear Ratio"
  Arm Secondary Encoders/1 -> Bus Creator1/6  "Has Secondary Enc"
  Arm robot type/1 -> Bus Creator4/1, Bus Creator6/2, decode robot/2(robot_type)  "robot type"
  Arm Torque Constant/1 -> Bus Creator4/2, Bus Creator6/4  "torque constant"
  Arm L5/1 -> Bus Creator4/3  "L5"
  Arm L2 L5 Angle/1 -> Bus Creator4/4  "L2L5 Angle"
  Bus Creator4/1 -> Bus Creator5/1
  Arm Force Sensor Angle Offset/1 -> Bus Creator4/5  "FT sensor angle"
  Arm Encoder Orientation 1/1 -> Bus Creator2/1  "Encoder 1 orientation"
  Arm Encoder Orientation 2/1 -> Bus Creator2/2  "Encoder 2 orientation"
  Bus Creator2/1 -> Bus Creator3/2
  Bus Creator3/1 -> pmac motor params/1
  Bus Creator5/1 -> hardware settings/1
  Bus Creator6/1 -> motor parameters/1
  Arm Shoulder Angle Offset/1 -> Bus Creator/1  "shoulder angle offset"
  Arm Elbow Angle Offset/1 -> Bus Creator/2  "elbow angle offset"
  Arm Shoulder X/1 -> Bus Creator/3  "Shoulder X"
  Arm Shoulder Y/1 -> Bus Creator/4  "Shoulder Y"
  Arm L1/1 -> Bus Creator/5  "L1"
  Arm L2/1 -> Bus Creator/6  "L2"
  Arm Pointer Offset/1 -> Bus Creator/7  "Pointer offset"
  Arm L3 Error/1 -> Bus Creator/8  "L3 Error"
  Bus Creator/1 -> calibration/1
  Bus Creator1/1 -> Bus Creator6/1, Bus Creator5/2, Bus Creator3/1  "R2"
  Arm robot version/1 -> Bus Creator5/3, Bus Creator6/3, decode robot/3(robot_version)  "robot version"
  [system_type] -> decode robot/1(system_type)
  decode robot/1(isEP) -> Bus Creator7/1  "isEP"
  decode robot/2(isHumanEXO) -> Bus Creator7/2  "isHumanExo"
  decode robot/3(isNHPEXO) -> Bus Creator7/3  "isNHPExo"
  decode robot/4(isClassicExo) -> Bus Creator7/4  "isClassicExo"
  decode robot/5(isUTSEXO) -> Bus Creator7/5  "isUTSExo"
  decode robot/6(isPMAC) -> Bus Creator7/6  "isPMAC"
  decode robot/7(isECAT) -> Bus Creator7/7  "isECAT"
  Bus Creator7/1 -> Bus Creator6/5  "R2Info"
  Status read1/1 -> Selector/1
  Selector/1 -> Bus Creator7/8  "robotRevision"

== system EMC_no_hand/DataLogging/Poll KINARM/constants/update constants subsystem ==
  Params : Inport
  Enable : EnablePort
  Arm Force Sensors : Constant  Value=[0 0]
  Bus Selector : BusSelector  OutputSignals=robot1 calibration params,robot2 calibration params
  Bus Selector1 : BusSelector  OutputSignals=robot1 hardware settings,robot2 hardware settings
  Bus to Vector{,1..3} (4 alike) : BusToVector
  Data Store Write : DataStoreWrite  DataStoreName=RobotCalibrations
  Data Store Write1 : DataStoreWrite  DataStoreName=HardwareSettings
  Data Store Write8 : DataStoreWrite  DataStoreName=ArmForceSensors
  Mux1 : Mux  Inputs=2
  Mux6 : Mux  Inputs=2
  wires:
  Mux6/1 -> Data Store Write/1
  Bus Selector/1 -> Bus to Vector/1  "<robot1 calibration params>"
  Bus Selector/2 -> Bus to Vector1/1  "<robot2 calibration params>"
  Mux1/1 -> Data Store Write1/1
  Params/1 -> Bus Selector1/1, Bus Selector/1
  Bus Selector1/1 -> Bus to Vector2/1  "<robot1 hardware settings>"
  Bus Selector1/2 -> Bus to Vector3/1  "<robot2 hardware settings>"
  Arm Force Sensors/1 -> Data Store Write8/1
  Bus to Vector/1 -> Mux6/1
  Bus to Vector1/1 -> Mux6/2
  Bus to Vector2/1 -> Mux1/1
  Bus to Vector3/1 -> Mux1/2

== system EMC_no_hand/DataLogging/Poll KINARM/createKINData/hand feedback ==
  note: The hand feedback settings here may or may not be used by the hand
      | feedback block, depending on its block mask settings. They are
      | transferred to the hand feedback block via the KINdata data structure.
  process_vcodes_requested_delay_s : Inport
  Gaze Feedback Status : Constant  Value=0
  Hand Feedback Colour : Constant  Value=16777215
  Hand Feedback Feed Forward : Constant  Value=.05
  Hand Feedback Radius : Constant  Value=0.005
  Hand Feedback Source : Constant  Value=0
  Hand Feedback Status : Constant  Value=3
  Mux5 : Mux  Inputs=7
  hand feedback settings : Outport
  wires:
  Gaze Feedback Status/1 -> Mux5/6
  Hand Feedback Colour/1 -> Mux5/4
  Hand Feedback Status/1 -> Mux5/1
  Hand Feedback Source/1 -> Mux5/2
  Mux5/1 -> hand feedback settings/1
  Hand Feedback Feed Forward/1 -> Mux5/5
  Hand Feedback Radius/1 -> Mux5/3
  process_vcodes_requested_delay_s/1 -> Mux5/7

== system EMC_no_hand/DataLogging/Poll KINARM/Force Sensor Control/Force Sensor 1 Subsystem/If Action Subsystem ==
  In1 : Inport
  Enable : EnablePort
  Byte Reversal : xpcutilitieslib/Byte Reversal   numInp=1
  Byte Reversal1 : xpcutilitieslib/Byte Reversal   numInp=1
  Byte Reversal2 : xpcutilitieslib/Byte Reversal   numInp=1
  Constant : Constant  Value=4660  OutDataTypeStr=uint16
  Constant1 : Constant  Value=0  OutDataTypeStr=uint32
  Constant2 : Constant  Value=0  OutDataTypeStr=uint16
  Constant3 : Constant  Value=2  OutDataTypeStr=uint16
  Pack : xpcobsoletelib/Utilities/Pack   datatypes={'uint16', 'uint16', 'uint32'}  byteAlign=1
  Send : xpcrtudplib/Legacy UDP/Send   ipAddress=192.168.0.10  ipPort=49152  localPort=51000  vblLen=on  sampletime=-1
  Switch : Switch  Criteria=u2 > Threshold
  Width : Width
  wires:
  In1/1 -> Switch/2
  Constant/1 -> Byte Reversal1/1
  Constant1/1 -> Byte Reversal2/1
  Constant3/1 -> Switch/1
  Constant2/1 -> Switch/3
  Switch/1 -> Byte Reversal/1
  Pack/1 -> Width/1, Send/1
  Byte Reversal1/1 -> Pack/1
  Byte Reversal/1 -> Pack/2
  Byte Reversal2/1 -> Pack/3
  Width/1 -> Send/2

== system EMC_no_hand/DataLogging/Poll KINARM/Force Sensor Control/Force Sensor 2 Subsystem/Data Transfer Start Subsystem ==
  In2 : Inport
  Enable : EnablePort
  Byte Reversal : xpcutilitieslib/Byte Reversal   numInp=1
  Byte Reversal1 : xpcutilitieslib/Byte Reversal   numInp=1
  Byte Reversal2 : xpcutilitieslib/Byte Reversal   numInp=1
  Constant : Constant  Value=4660  OutDataTypeStr=uint16
  Constant1 : Constant  Value=0  OutDataTypeStr=uint32
  Constant2 : Constant  Value=0  OutDataTypeStr=uint16
  Constant3 : Constant  Value=2  OutDataTypeStr=uint16
  Pack : xpcobsoletelib/Utilities/Pack   datatypes={'uint16', 'uint16', 'uint32'}  byteAlign=1
  Send : xpcrtudplib/Legacy UDP/Send   ipAddress=192.168.0.11  ipPort=49152  localPort=51001  vblLen=on  sampletime=-1
  Switch : Switch  Criteria=u2 > Threshold
  Width : Width
  wires:
  In2/1 -> Switch/2
  Constant/1 -> Byte Reversal1/1
  Constant1/1 -> Byte Reversal/1
  Constant3/1 -> Switch/1
  Constant2/1 -> Switch/3
  Switch/1 -> Byte Reversal2/1
  Pack/1 -> Width/1, Send/1
  Byte Reversal/1 -> Pack/3
  Byte Reversal1/1 -> Pack/1
  Byte Reversal2/1 -> Pack/2
  Width/1 -> Send/2

== system EMC_no_hand/DataLogging/Poll KINARM/PMAC Subsystem/read_pmac/DPRAM Access Subsystem ==
  note: This PMAC needs a 16-bit integer for the watchdog input, but writemem
      | only writes singles.  So we need to typecast to single first
  note: This subsystem provides BKIN client software with access to the DPRAM of the motion control card.
      |
      | To read a value from DPRAM: write the value's offset to DPRAMReadOffset, set the switch indicating
      | whether the address holds a floating or fixed point value, then set the read switch high and allow the
      | result to propagate. Read the value, stored as a double, from DPRAMReadValue.
      |
      | To write a value to DPRAM: write the value to DPRAMWriteValue and its offset to DPRAMWriteOffset,
      | set the write switch high, and then allow the result to propagate. There is currently no option to write
      | values as UInt32s, akin to that for reading values.
      |
      | The default value for the offsets (0x216) is the lowest meaningful offset, the PLC switch variable.
  Counter Free-Running : simulink/Sources/Counter Free-Running  NumBits=16  tsamp=-1
  DPRAM Read Offset : Constant  Value=534  OutDataTypeStr=double
  DPRAM Read Value : Gain  SaturateOnIntegerOverflow=on  OutDataTypeStr=Inherit: Same as input  ParamDataTypeStr=Inherit: Same as input
  DPRAM WatchDog offset : Constant  Value=627  OutDataTypeStr=double
  DPRAM Write Offset : Constant  Value=534  OutDataTypeStr=double
  DPRAM Write Value : Constant
  Data Type Conversion : DataTypeConversion  OutDataTypeStr=uint32  SaturateOnIntegerOverflow=on  RndMeth=Zero
  If : If  NumInputs=2  IfExpression=u2 > u1  ShowElse=off
  If1 : If  NumInputs=2  IfExpression=u2 > u1  ShowElse=off
  Read DPRAM : Subsystem  TreatAsAtomicUnit=on
  Read Switch : Constant  Value=0
  Read as UInt32 : Constant  Value=0  OutDataTypeStr=double
  Terminator : Terminator
  TypeCast : MATLAB Function  TreatAsAtomicUnit=on
  Unit Delay : UnitDelay  SampleTime=-1
  Unit Delay1 : UnitDelay  SampleTime=-1
  Write : S-Function  Priority=6  FunctionName=mcc_writemem
  Write DPRAM : Subsystem  TreatAsAtomicUnit=on
  Write Switch : Constant  Value=0
  wires:
  TypeCast/1(y) -> Write/2
  DPRAM Write Offset/1 -> Write DPRAM/1(offset)
  DPRAM Write Value/1 -> Write DPRAM/2(value)
  If1/1 -> Write DPRAM/Action
  Write Switch/1 -> Unit Delay1/1, If1/2
  DPRAM Read Value/1 -> Terminator/1
  Read DPRAM/1(result) -> DPRAM Read Value/1
  If/1 -> Read DPRAM/Action
  DPRAM Read Offset/1 -> Read DPRAM/1(offset)
  Read Switch/1 -> Unit Delay/1, If/2
  Unit Delay/1 -> If/1
  Unit Delay1/1 -> If1/1
  Read as UInt32/1 -> Read DPRAM/2(read as uint32)
  Data Type Conversion/1 -> Write/1
  DPRAM WatchDog offset/1 -> Data Type Conversion/1
  Counter Free-Running/1 -> TypeCast/1(u)

== system EMC_no_hand/DataLogging/Poll KINARM/PMAC Subsystem/read_pmac/DPRAM Access Subsystem/Read DPRAM ==
  offset : Inport
  read as uint32 : Inport  Port=2
  Action Port : ActionPort  ActionType=then
  Data Type Conversion : DataTypeConversion  OutDataTypeStr=uint32  SaturateOnIntegerOverflow=on  RndMeth=Zero
  Data Type Conversion1 : DataTypeConversion  OutDataTypeStr=double  SaturateOnIntegerOverflow=on  RndMeth=Zero
  Data Type Conversion2 : DataTypeConversion  OutDataTypeStr=uint32  SaturateOnIntegerOverflow=on  RndMeth=Zero
  Mux : Mux  Inputs=2
  Read : S-Function  Priority=6  FunctionName=mcc_readmem
  result : Outport
  wires:
  Data Type Conversion/1 -> Mux/1
  Data Type Conversion1/1 -> result/1
  Read/1 -> Data Type Conversion1/1
  offset/1 -> Data Type Conversion/1
  read as uint32/1 -> Data Type Conversion2/1
  Data Type Conversion2/1 -> Mux/2
  Mux/1 -> Read/1

== system EMC_no_hand/DataLogging/Poll KINARM/PMAC Subsystem/read_pmac/DPRAM Access Subsystem/Write DPRAM ==
  offset : Inport
  value : Inport  Port=2
  Action Port : ActionPort  ActionType=then
  Data Type Conversion : DataTypeConversion  OutDataTypeStr=uint32  SaturateOnIntegerOverflow=on  RndMeth=Zero
  Data Type Conversion1 : DataTypeConversion  OutDataTypeStr=single  SaturateOnIntegerOverflow=on  RndMeth=Zero
  Write : S-Function  Priority=6  FunctionName=mcc_writemem
  wires:
  Data Type Conversion1/1 -> Write/2
  Data Type Conversion/1 -> Write/1
  offset/1 -> Data Type Conversion/1
  value/1 -> Data Type Conversion1/1

== matlab function EMC_no_hand/Target state & position data/MATLAB Function1 ==
  data: targetVCode input; targetOn output; targetX output; targetY output
%This function extracts data to be saved from the target VCode matrix
%(includes both circle & both ellipse targets, not the start target/fixation cross or hand feedback) 
%Returns a vector of doubles.
%VCode order: first circle, first ellipse, second circle, second ellipse
function [targetOn, targetX, targetY] = extractDataChannels(targetVCode)
%#codegen
    onOff = targetVCode(2);
    onOff = typecast(onOff, 'double');
    xPosition = targetVCode(3);
    xPosition = typecast(xPosition, 'double');
    yPosition = targetVCode(4);
    yPosition = typecast(yPosition, 'double');
    
    targetOn = onOff;
    targetX = xPosition;
    targetY = yPosition;
end

== stateflow chart EMC_no_hand/Trial Control ==
  state Initialiize/
    entry: trial_start_trigger = 0;
    trial_in_progress = 0;
    target_state = 0;
    movement_delay = Task_Wide_Parameters[MOVEMENT_DELAY];//Already in ms
    post_trial_delay = Task_Wide_Parameters[POST_TRIAL_DELAY];//Already in ms
    path_time = Task_Wide_Parameters[PATH_PERIOD] * 1000;//Convert to ms
    event_code = 0;
    trial_start_trigger = 1;
    force_on = 0
  state MainTrial
    state Start/
      target_state = 1;
      event_code = TRIAL_START;
    state SeekingFixation/
      event_code = DETECT_FIXATION;
      state GazeNotInTarget/
      state GazeInTarget/
        event_code = GAZE_IN_TARGET;
      (default) -> GazeNotInTarget
      GazeNotInTarget -> GazeInTarget : //gaze enters cross region
          | [gaze_in_target == 1]
      GazeInTarget -> GazeNotInTarget [order 2] : //gaze exits cross region
          | [gaze_in_target == 0 && angular_velocity > Task_Wide_Parameters[ANGULAR_THRESHOLD]]/event_code = GAZE_EXIT;
    state TriggerOn/
      trial_start_trigger = 1;
    state TriggerOff/
      entry: trial_start_trigger = 0;
    state TrialInProgress/
      entry: trial_in_progress = 1;
      force_on = 1;
      event_code = TRIAL_MOVEMENT;
    state End/
      entry: trial_in_progress = 0;
      event_code = TRIAL_END;
    Start -> SeekingFixation : // has the hand remained stable for the specified amount of time?
        | after(Task_Wide_Parameters[START_STABILIZATION],e_clk)
    GazeInTarget -> TriggerOn [order 1] : after(Task_Wide_Parameters[FIXATION_DURATION], e_clk)
    TriggerOn -> TriggerOff : after(1,e_clk)
    TriggerOff -> TrialInProgress : after(movement_delay, e_clk)
    TrialInProgress -> End : after(path_time, e_clk)
  state Inter_Trial_State/
    // Turn off targets and force, reset the event code, and send the
    //e_Trial_End Stateflow event to indicate that the trial is over.
    entry: target_state = 0;
    force_on = 0;
    event_code = TRIAL_RESET;
    e_Trial_End;
  (default) -> Initialiize
  Initialiize -> Start
  Inter_Trial_State -> Start : // Proceed after post-trial delay
      | after(post_trial_delay, e_clk)
  MainTrial -> Inter_Trial_State : e_ExitTrialNow/
      | // e_ExitTrialNow event occurs if the
      | // Dex pause is pressed by the operator
  End -> Inter_Trial_State
  data: Task_Wide_Parameters input double; event_code output uint16 [0..] =0; trial_start_trigger output boolean; post_trial_delay local double; movement_delay local double; path_time local double; target_state output int8; trial_in_progress output double; gaze_in_target input boolean; angular_velocity input double; hand_in_target input boolean; force_on output boolean
  events: e_clk input RISING_EDGE_EVENT; e_ExitTrialNow input EITHER_EDGE_EVENT; e_Trial_End output EITHER_EDGE_EVENT

== matlab function EMC_no_hand/Position function/MATLAB Function ==
  data: pseudorandom_trajectory_parameters output; diagonal_trajectory_parameters output; sinusoidal_trajectory_parameters output
function [pseudorandom_trajectory_parameters, diagonal_trajectory_parameters, sinusoidal_trajectory_parameters] = generate_parameter_tables()
    %#codegen
    %Pseudorandom Trajectory Parameter Table Key:
    %Row 1: A1x
    %Row 2: A2x
    %Row 3: Harmonic x
    %Row 4: Phase x (degrees)
    %Row 5: A1y
    %Row 6: A2y
    %Row 7: Harmonic y
    %Row 8: Phase y (degrees)
    pseudorandom_trajectory_parameters = [5,4,4,5,5.1;5,5,5.1,5,5.2;2,2,3,3,2;45,-60,-60,90,-90;5,3,4,3.4,4;5,5,5.2,5,5;3,3,2,2,3;-135,-135,-135,45,22.5];
    
    %Note: This matrix is formulated in (columns, rows) and then transposed
    %Diagonal Trajectory Parameter Table Key:
    %Row 1: Theta (displacement from 0 radians of line)
    %Row 2: Horizontal direction (-1 left, 1 right)
    %Row 3: Vertical direction (-1 down, 1 up)
    diagonal_trajectory_parameters = [15,-1,-1;15,-1,1;15,1,-1;15,1,1;30,-1,-1;30,-1,1;30,1,-1;30,1,1;45,-1,-1;45,-1,1;45,1,-1;45,1,1;60,-1,-1;60,-1,1;60,1,-1;60,1,1;75,-1,-1;75,-1,1;75,1,-1;75,1,1].';
    
    %Note: This matrix is formulated in (columns, rows) and then transposed
    %Sinusoidal Trajectory Parameter Table Key:
    %Row 1: Frequency: Number of waves (full oscillations) per meter
    %Row 2: Horizontal direction (-1 left, 1 right)
    %Row 3: Vertical direction (-1 down, 1 up)
    sinusoidal_trajectory_parameters = [5,-1,-1;5,-1,1;5,1,-1;5,1,1;10,-1,-1;10,-1,1;10,1,-1;10,1,1;15,-1,-1;15,-1,1;15,1,-1;15,1,1;20,-1,-1;20,-1,1;20,1,-1;20,1,1;25,-1,-1;25,-1,1;25,1,-1;25,1,1].';
end

== matlab function EMC_no_hand/Angular  velocity calculation/Gaze angular velocity ==
  data: gazeData input; angularVelocity output
function angularVelocity = getAngularVelocity(gazeData)
    %#codegen
    %TODO: Correct for delay
    height = 0.22;
    persistent gazeXYZ timestamp; %seconds
    if isempty(gazeXYZ)
        gazeXYZ = [0 0 height];
    end
    if isempty(timestamp)
        timestamp = 0;
    end
    newXYZ = [gazeData(1), gazeData(2), height];
    if timestamp ~= 0
        angleChange = (180 / pi) * atan2(norm(cross(newXYZ,gazeXYZ)),dot(newXYZ,gazeXYZ)); %alternate methods for computing this angle using trig?
    else
        angleChange = -100; %code to prevent skewed results from first iteration
    end
    newTimestamp = gazeData(3);
    timestampChange = newTimestamp - timestamp;
    gazeXYZ = newXYZ;
    timestamp = newTimestamp;
    angularVelocity = angleChange / timestampChange;
end

== matlab function EMC_no_hand/Chk Gaze in Target/MATLAB Function ==
  data: gaze input; gaze_in_target output; target input; dist output; logical_radius input
function [gaze_in_target,dist] = gazeInTargetCheck(gaze,target, logical_radius)
%#codegen

gazex=gaze(1); %Hand Coordinates X and Y
gazey=gaze(2);

targetx=target(3);  %coordinates of center in m. 
targety=target(4);
%radius=target(5);

dist=sqrt((gazex-targetx)^2+(gazey-targety)^2);

if dist<=logical_radius 
    gaze_in_target=1;
else
    gaze_in_target=0;
end
